simulink model "Final_Project_Arrangement"  (R2018b)
settings: Solver=VariableStepAuto  StartTime=0.0  StopTime=0.1  RelTol=1e-3
undefined symbols (not defined in the file): Ion, Lithium
libraries: powerlib x13, electricdrivelib x1, spsDrivesDcBusModel x1, re_lib x1
settings Model: Creator=Vishant  LastModifiedBy=Vishant

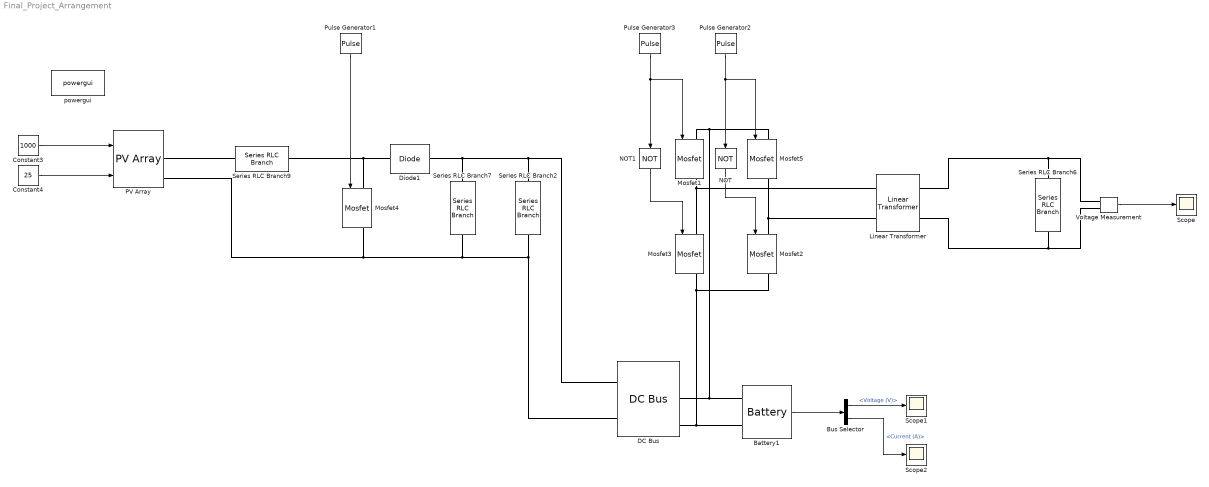
== system Final_Project_Arrangement ==
  Battery1 : electricdrivelib/Extra Sources/Battery  BatType=Lithium-Ion  ShowTempParam=off  ThermalPreset=no  ShowAgeParam=off  NomV=48  NomQ=100  SOC=5  Batt_Tr=30  PresetModel=on  MaxQ=100  MinV=36  FullV=55.8714  Dis_rate=43.4783  R=0.0048  Normal_OP=90.4348  expZone="[51.8585      4.91304]"  current=[6.5 13 32.5]  Units=Time  Tci=20  NomT=20  T2=-30  MaxQ2=4.8  FullV2=7.1  Normal_OP2=5.655  expZone2="[6.58           1]"  Rca=0.6  ti=2000  Dp=0  Neq0=0  Tsim=1e6  Ta1=25  Qeol=5.4*0.9  Reol=0.013333*1.2  Char_age=[2.3478, 3]  Dis_age=[2.3478, 10]  N1=1500  N2=10500  N3=1000  N4=1400  Ta2=45  N5=950
  Bus Selector : BusSelector  OutputSignals=Voltage (V),Current (A)
  Constant3 : Constant  Value=1000
  Constant4 : Constant  Value=25
  DC Bus : spsDrivesDcBusModel/DC Bus   busType=Capacitive (generic)  Ts=2e-6  capacitance=2000e-6  inductance=1e-3  Setx0=off  InitialVoltage=600  Rbrake=8  frequency=4000  activationVoltage=320  shutdownVoltage=310
      settings: SourceProductName=The database C:\Users\ak23510\AppData\Roaming\MathWorks\MATLAB\R2017a\slblocks_master.db is locked, or a table in the database is locked. (database is locked)
  Diode1 : powerlib/Power Electronics/Diode  Ron=1e-9  Lon=0  Vf=0  IC=0  UseSnubber=0  Rs=inf  Cs=0  Measurements=off
  Linear Transformer : powerlib/Elements/Linear Transformer  UNITS=SI  NominalPower=[ 240 50 ]  winding1=[230/7 0 0]  winding2=[237.58 0 0]  ThreeWindings=off  winding3=[3.15e+05 8.2688e+05 1.0528e+05]  RmLm=[Inf 10e-3]  Measurements=None  DataType=on
  Mosfet{1..5} (5 alike) : powerlib/Power Electronics/Mosfet  Ron=1e-9  Lon=0  Rd=0  Vfd=0  IC=0  Rs=inf  Cs=0  Measurements=on
  NOT : Logic  Operator=NOT  IconShape=distinctive  AllPortsSameDT=off  OutDataTypeStr=boolean
  NOT1 : Logic  Operator=NOT  IconShape=distinctive  AllPortsSameDT=off  OutDataTypeStr=boolean
  PV Array : re_lib/Solar/PV Array  Npar=1  Nser=1  PlotType=one module @ 25 deg.C & specified irradiances  S_vec="[ 1000  500  100 ]"  Temp_C_vec=[ 1000 500 100 ]  ModuleName=User-defined  PlotWhenSelected=off  Pm=260.0665  Ncell=60  Voc=39.10  Isc=8.56  Vm=31.91  Im=8.15  beta_Voc_pc=-0.33  alpha_Isc_pc=0.06  beta_Voc=-0.12903  alpha_Isc=0.005136  IL=8.6323  I0=9.8374e-11  nI=1.0071  Rsh=405.3185  Rs=0.31166  BAL=off  Tc=1e-10  Tfilter=5e-5
  Pulse Generator1 : DiscretePulseGenerator  PulseType=Time based  Period=1/100000  PulseWidth=33
  Pulse Generator2 : DiscretePulseGenerator  PulseType=Time based  Period=1/50  PulseWidth=50  PhaseDelay=0.0047
  Pulse Generator3 : DiscretePulseGenerator  PulseType=Time based  Period=1/50  PulseWidth=50
  Scope : Scope
  Scope1 : Scope
  Scope2 : Scope
  Series RLC Branch2 : powerlib/Elements/Series RLC Branch  LConnTagsString=__new0  RConnTagsString=__new0  BranchType=R  Resistance=8.86  Inductance=1e-3  SetiL0=off  InitialCurrent=0  Capacitance=1e-6  Setx0=off  InitialVoltage=0  Measurements=None
  Series RLC Branch6 : powerlib/Elements/Series RLC Branch  LConnTagsString=__new0  RConnTagsString=__new0  BranchType=R  Resistance=8.86  Inductance=1e-3  SetiL0=off  InitialCurrent=0  Capacitance=1e-6  Setx0=off  InitialVoltage=0  Measurements=None
  Series RLC Branch7 : powerlib/Elements/Series RLC Branch  LConnTagsString=__new0  RConnTagsString=__new0  BranchType=C  Resistance=1  Inductance=1e-3  SetiL0=off  InitialCurrent=0  Capacitance=18e-6  Setx0=off  InitialVoltage=0  Measurements=None
  Series RLC Branch9 : powerlib/Elements/Series RLC Branch  LConnTagsString=__new0  RConnTagsString=__new0  BranchType=L  Resistance=1  Inductance=50e-6  SetiL0=off  InitialCurrent=0  Capacitance=1e-6  Setx0=off  InitialVoltage=0  Measurements=None
  Voltage Measurement : powerlib/Measurements/Voltage Measurement  PhasorSimulation=off  OutputType=Complex  PSBequivalent=0
  powergui : powerlib/powergui  Priority=1  SimulationMode=Continuous  SampleTime=50e-6  frequency=60  Iterations=50  frequencyindice=0  Pbase=100e6  ErrMax=1e-4  UnitsV=kV  UnitsW=MW  buscounter=0  FunctionMessages=off  echomessages=off  EnableUseOfTLC=off  CurrentSourceSwitches=off  DisableSnubberDevices=off  DisableRonSwitches=off  DisableVfSwitches=off  DisplayEquations=off  SolverType=Tustin/Backward Euler (TBE)  Interpol=off  ExternalGateDelay=off  methode=off  Ts=100  x0status=blocks  SPID=on  SwTol=0  HookPort=off  RestoreLinks=warning  ResistiveCurrentMeasurement=off  Frange=[0:2:500]  Ylog=off  Xlog=on  ShowGrid=off  save=off  variable=ZData  structure=0  ZoomFFT=off  StartTime=0.0  cycles=1  DisplayStyle=1  fundamental=60  FreqAxis=off  MaxFrequency=1000  frequencyindicesteady=1  RmsSteady=1  display=off
  wires:
  Constant4/1 -> PV Array/2
  Constant3/1 -> PV Array/1
  Pulse Generator2/1 -> Mosfet5/1, NOT/1
  Pulse Generator3/1 -> Mosfet1/1, NOT1/1
  Pulse Generator1/1 -> Mosfet4/1
  NOT1/1 -> Mosfet3/1
  NOT/1 -> Mosfet2/1
  Voltage Measurement/1 -> Scope/1
  Battery1/1 -> Bus Selector/1
  Bus Selector/1 -> Scope1/1  "<Voltage (V)>"
  Bus Selector/2 -> Scope2/1  "<Current (A)>"
  connections:
  Linear Transformer/LConn1 -- Mosfet3/LConn1 -- Mosfet1/RConn1
  Series RLC Branch7/RConn1 -- DC Bus/LConn2 -- Series RLC Branch2/RConn1 -- Mosfet4/RConn1 -- PV Array/RConn2
  Series RLC Branch7/LConn1 -- Series RLC Branch2/LConn1 -- DC Bus/LConn1 -- Diode1/RConn1
  Diode1/LConn1 -- Series RLC Branch9/RConn1 -- Mosfet4/LConn1
  PV Array/RConn1 -- Series RLC Branch9/LConn1
  Series RLC Branch6/LConn1 -- Voltage Measurement/LConn1 -- Linear Transformer/RConn1
  Series RLC Branch6/RConn1 -- Voltage Measurement/LConn2 -- Linear Transformer/RConn2
  Linear Transformer/LConn2 -- Mosfet5/RConn1 -- Mosfet2/LConn1
  Battery1/LConn1 -- Mosfet1/LConn1 -- Mosfet5/LConn1 -- DC Bus/RConn1
  Mosfet2/RConn1 -- Battery1/LConn2 -- DC Bus/RConn2 -- Mosfet3/RConn1
